simulink subsystem "HEVIPSSSC"  (R2025b)
settings: Solver=VariableStepAuto  StartTime=0.0  StopTime=10.0  RelTol=1e-3
undefined symbols (not defined in the file): EM1, EM2, PlntHevIpsP1CarrDamp, PlntHevIpsP1PlanetDamp, PlntHevIpsP1RingDamp, PlntHevIpsP1SunDamp, PlntHevIpsP1SunRingRatio, PlntHevIpsP2InDamp, PlntHevIpsP2OutDamp
libraries: fl_lib x7, sdl_lib x2
settings Model: ModifiedByFormat=The MathWorks, Inc.  Creator=The MathWorks, Inc.  LastModifiedBy=The MathWorks, Inc.
settings OptimizationCC: ReuseModelBlockBuffer=off
settings DebuggingCC: SubsystemReferenceDiagnosticForUnitTest=warning
settings RTWCC: GPUComputeCapability=3.5

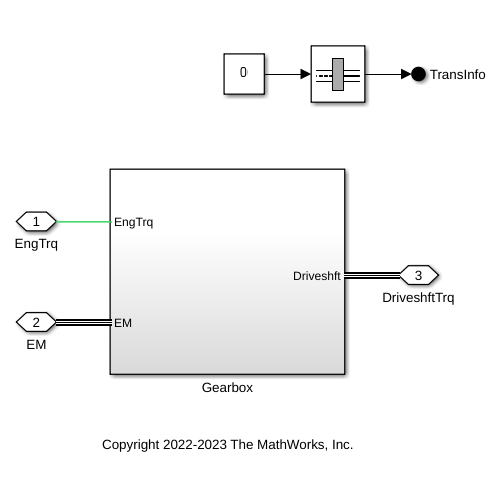
[thumbnail: Simulink's stored preview of the top-level diagram]
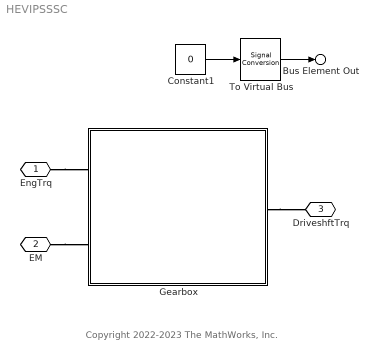
== system HEVIPSSSC ==
  note: Copyright 2022-2023 The MathWorks, Inc.
  Constant1 : Constant  Value=0  OutDataTypeStr=Bus: TransInfoBUS  SampleTime=Inf
  Gearbox : Subsystem  VariantControl=Simscape
  To Virtual Bus : SignalConversion  ConversionOutput=Virtual bus  OverrideOpt=off
  EngTrq : PMIOPort  Side=Left
  EM : PMIOPort  Port=2  Side=Left
  DriveshftTrq : PMIOPort  Port=3  Side=Right
  Bus Element Out : Outport  PortName=TransInfo
  wires:
  Constant1/1 -> To Virtual Bus/1
  To Virtual Bus/1 -> Bus Element Out/1
  connections:
  EM/RConn1 -- Gearbox/LConn2
  Gearbox/RConn1 -- DriveshftTrq/RConn1
  EngTrq/RConn1 -- Gearbox/LConn1

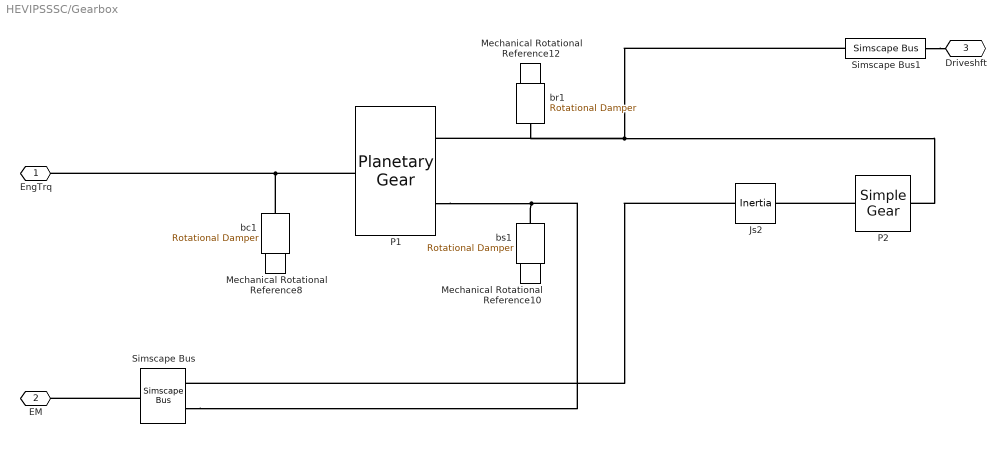
== system HEVIPSSSC/Gearbox ==
  Js2 : fl_lib/Mechanical/Rotational Elements/Inertia  inertia=PlntHevIpsP2InInertia kg*m^2  num_ports=foundation.enum.numPorts2.two  w_specify=on  w_priority=High  w=0 rad/s  w_nominal_specify=off  w_nominal_value=1  w_nominal_unit=rad/s  t_specify=off  t_priority=None  t=0 N*m  t_nominal_specify=off  t_nominal_value=1  t_nominal_unit=N*m
      settings: InternalSimscapePortConfiguration="{\"Bottom\":[],\"Left\":[{\"id\":\"I\",\"label\":\"\",\"type\":\"foundation.mechanical.rotational.rotational\"}],\"Right\":[{\"id\":\"J\",\"label\":\"\",\"type\":\"foundation.mechanical.rotational.rotational\"}],\"Top\":[]}"
  Mechanical Rotational Reference10 : fl_lib/Mechanical/Rotational Elements/Mechanical Rotational Reference
  Mechanical Rotational Reference12 : fl_lib/Mechanical/Rotational Elements/Mechanical Rotational Reference
  Mechanical Rotational Reference8 : fl_lib/Mechanical/Rotational Elements/Mechanical Rotational Reference
  P1 : sdl_lib/Gears/Planetary Gear  rs_ratio=1/PlntHevIpsP1SunRingRatio  friction_model=sdl.enum.gear_friction.constant  efficiency=PlntHevIpsP1GearEff  temperature_TLU=[ 280 300 320 ] K  efficiency_sp_TLU=[ 0.95 0.9 0.85 ]  efficiency_rp_TLU=[ 0.95 0.9 0.85 ]  pwr_thr=PlntHevIpsP1GearPwrThresh W  mu_visc=[0 PlntHevIpsP1PlanetDamp] N*m/(rad/s)  model_inertia=1  sun_inertia=PlntHevIpsP1SunInertia kg*m^2  ring_inertia=PlntHevIpsP1RingInertia kg*m^2  carrier_inertia=PlntHevIpsP1CarrInertia kg*m^2  carrier_radius=PlntHevIpsP1CarrRadius m  planet_inertia=PlntHevIpsP1PlanetInertia kg*m^2  planet_mass=PlntHevIpsP1PlanetMass kg  thermal_mass=50 J/K  T_init=300 K
      settings: LogSimulationData=on
  P2 : sdl_lib/Gears/Simple Gear  ratio=PlntHevIpsP2GearRatio  rotation_direction=sdl.enum.shaftOutputDirection.same  friction_model=sdl.enum.gear_efficiencies_load.constant  T_noload=0.1 N*m  T_nom=5 N*m  efficiency_nom=0.8  efficiency=PlntHevIpsP2Eff  temperature_TLU=[280, 300, 320] K  load_TLU=[1, 5, 10] N*m  efficiency_TLU=[.95, .9, .85]  efficiency_TLU2=[.85, .8, .75; .95, .9, .85; .85, .8, .7]  w_thr=0.01 rad/s  pwr_thr=PlntHevIpsP2PwrThresh W  enable_backlash=false  hardstop_model=simscape.enum.hardstop.smooth  backlash_distance=1e-3 mm  r_base=0.1 m  transition=1e-4 mm  backlash_stiffness=1e7 N/m  backlash_damping=1e6 N*s/m  coeff_rest=0.7  v_tol=0.001 m/s  f_tol=0.001 N  mu_visc=[PlntHevIpsP2InDamp, PlntHevIpsP2OutDamp] N*m*s/rad  thermal_mass=50 J/K  temperature_specify=off  temperature_priority=High  temperature=300 K  temperature_nominal_specify=off  temperature_nominal_value=1  temperature_nominal_unit=K  x_backlash_specify=off  x_backlash_priority=None  x_backlash=0 mm  x_backlash_nominal_specify=off  x_backlash_nominal_value=1  x_backlash_nominal_unit=mm  f_hardstop_specify=off  f_hardstop_priority=None  f_hardstop=0 N  f_hardstop_nominal_specify=off  f_hardstop_nominal_value=1  f_hardstop_nominal_unit=N  v_backlash_specify=off  v_backlash_priority=None  v_backlash=0 m/s  v_backlash_nominal_specify=off  v_backlash_nominal_value=1  v_backlash_nominal_unit=m/s
  Simscape Bus : SimscapeBus  HierarchyStrings=EM1;EM2
  Simscape Bus1 : SimscapeBus  HierarchyStrings=DriveshftTrq1
  bc1 : fl_lib/Mechanical/Rotational Elements/Rotational Damper  D=PlntHevIpsP1CarrDamp N*m/(rad/s)  w_specify=on  w_priority=High  w=0 rad/s  w_nominal_specify=off  w_nominal_value=1  w_nominal_unit=rad/s  t_specify=off  t_priority=None  t=0 N*m  t_nominal_specify=off  t_nominal_value=1  t_nominal_unit=N*m
  br1 : fl_lib/Mechanical/Rotational Elements/Rotational Damper  D=PlntHevIpsP1RingDamp N*m/(rad/s)  w_specify=on  w_priority=High  w=0 rad/s  w_nominal_specify=off  w_nominal_value=1  w_nominal_unit=rad/s  t_specify=off  t_priority=None  t=0 N*m  t_nominal_specify=off  t_nominal_value=1  t_nominal_unit=N*m
  bs1 : fl_lib/Mechanical/Rotational Elements/Rotational Damper  D=PlntHevIpsP1SunDamp N*m/(rad/s)  w_specify=on  w_priority=High  w=0 rad/s  w_nominal_specify=off  w_nominal_value=1  w_nominal_unit=rad/s  t_specify=off  t_priority=None  t=0 N*m  t_nominal_specify=off  t_nominal_value=1  t_nominal_unit=N*m
  EngTrq : PMIOPort  Side=Left
  EM : PMIOPort  Port=2  Side=Left
  Driveshft : PMIOPort  Port=3  Side=Right
  connections:
  bc1/LConn1 -- Mechanical Rotational Reference8/LConn1
  bs1/LConn1 -- Mechanical Rotational Reference10/LConn1
  br1/LConn1 -- Mechanical Rotational Reference12/LConn1
  bc1/RConn1 -- P1/LConn1 -- EngTrq/RConn1
  P2/LConn1 -- Js2/LConn1
  Simscape Bus1/LConn1 -- P2/RConn1 -- P1/RConn1 -- br1/RConn1
  Simscape Bus/RConn1 -- EM/RConn1
  Simscape Bus1/RConn1 -- Driveshft/RConn1
  Js2/RConn1 -- Simscape Bus/LConn1
  bs1/RConn1 -- P1/RConn2 -- Simscape Bus/LConn2
